simulink model "Original_TankSim_Model"  (R2024b)
settings: Solver=VariableStepAuto  StartTime=0.0  StopTime=1000  RelTol=1e-3
settings Model: Creator=carlo  LastModifiedBy=carlo

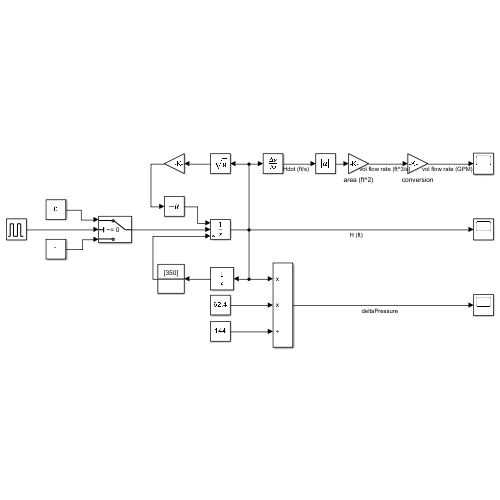
[thumbnail: Simulink's stored preview of the top-level diagram]
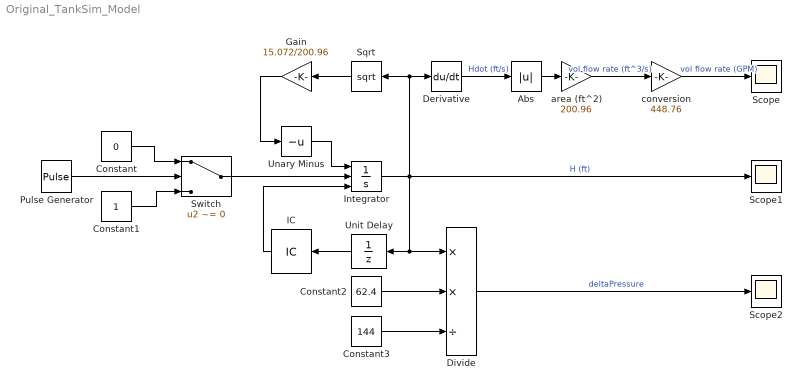
== system Original_TankSim_Model ==
  Abs : Abs  SaturateOnIntegerOverflow=off
  Constant : Constant  Value=0
  Constant1 : Constant
  Constant2 : Constant  Value=62.4
  Constant3 : Constant  Value=144
  Derivative : Derivative
  Divide : Product  Inputs=**/
  Gain : Gain  Gain=15.072/200.96
  IC : InitialCondition  Value=350
  Integrator : Integrator  ExternalReset=level hold  InitialConditionSource=external
  Pulse Generator : DiscretePulseGenerator  PulseType=Time based  Period=500  PulseWidth=50  PhaseDelay=300
  Scope : Scope
  Scope1 : Scope
  Scope2 : Scope
  Sqrt : Sqrt
  Switch : Switch  Criteria=u2 ~= 0  SaturateOnIntegerOverflow=off  InputSameDT=off
  Unary Minus : UnaryMinus
  Unit Delay : UnitDelay  SampleTime=-1  HasFrameUpgradeWarning=on
  area (ft^2) : Gain  Gain=200.96
  conversion : Gain  Gain=448.76
  wires:
  area (ft^2)/1 -> conversion/1  "vol flow rate (ft^3/s)"
  Derivative/1 -> Abs/1  "Hdot (ft/s)"
  Integrator/1 -> Scope1/1, Derivative/1, Sqrt/1, Divide/1, Unit Delay/1  "H (ft)"
  Unary Minus/1 -> Integrator/1
  Gain/1 -> Unary Minus/1
  Switch/1 -> Integrator/2
  Sqrt/1 -> Gain/1
  Unit Delay/1 -> IC/1
  IC/1 -> Integrator/3
  conversion/1 -> Scope/1  "vol flow rate (GPM)"
  Constant2/1 -> Divide/2
  Constant3/1 -> Divide/3
  Constant1/1 -> Switch/3
  Constant/1 -> Switch/1
  Pulse Generator/1 -> Switch/2
  Divide/1 -> Scope2/1  "deltaPressure"
  Abs/1 -> area (ft^2)/1
